simulink model "CryoDetMultiChan_CMB"  (R2016b)
settings: Solver=ode45  StartTime=0.0  StopTime=400e-6  MaxStep=Tclk/4  RelTol=1e-3
values from neighbouring files (symbols this model uses):
  ds_axi = 16    [setupCryoFPGA_CMB.m]
  Fclk = Fadc    (= 307200000)    [setupCryoFPGA_CMB.m]
  lpf = tf(num,den)    [setupCryoFPGA_CMB.m]
  Tclk = 1/Fclk    (= 3.25520833333e-09)    [setupCryoFPGA_CMB.m]
  Ts = 1/Fs    (= 3.25520833333e-09)    [setupADCtoDACloopback.m]    (also in setupCryoFPGA_CMB.m)
undefined symbols (not defined in the file or in its folder): AXI4, i, Lite, xlipgetpartsetting
libraries: xbsIndex_r4 x2215, hdlsllib x6, simulink x3, CryoDetLib x2
(part 4 of 16)

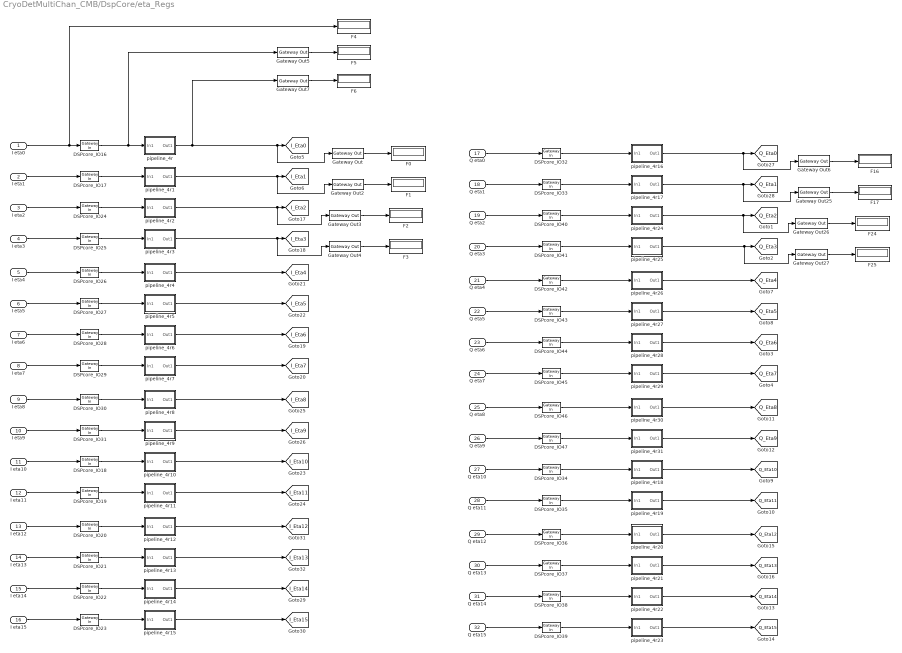
== system CryoDetMultiChan_CMB/DspCore/eta_Regs ==
  "I eta0 " : Inport
  I eta1 : Inport  Port=2
  I eta2 : Inport  Port=3
  I eta3 : Inport  Port=4
  I eta4 : Inport  Port=5
  I eta5 : Inport  Port=6
  I eta6 : Inport  Port=7
  I eta7 : Inport  Port=8
  I eta8 : Inport  Port=9
  I eta9 : Inport  Port=10
  I eta10 : Inport  Port=11
  I eta11 : Inport  Port=12
  I eta12 : Inport  Port=13
  I eta13 : Inport  Port=14
  I eta14 : Inport  Port=15
  I eta15 : Inport  Port=16
  Q eta0 : Inport  Port=17
  Q eta1 : Inport  Port=18
  Q eta2 : Inport  Port=19
  Q eta3 : Inport  Port=20
  Q eta4 : Inport  Port=21
  Q eta5 : Inport  Port=22
  Q eta6 : Inport  Port=23
  Q eta7 : Inport  Port=24
  Q eta8 : Inport  Port=25
  Q eta9 : Inport  Port=26
  Q eta10 : Inport  Port=27
  Q eta11 : Inport  Port=28
  Q eta12 : Inport  Port=29
  Q eta13 : Inport  Port=30
  Q eta14 : Inport  Port=31
  Q eta15 : Inport  Port=32
  DSPcore_IO16 : xbsIndex_r4/Gateway In  gui_display_data_type=Fixed-point  arith_type="Signed  (2's comp)"  n_bits=32  bin_pt=31  preci_type=Single  exp_width=8  frac_width=24  rows=1  columns=1  quantization=Truncate  overflow=Wrap  period=Tclk*ds_axi  UseAsADC=off  ADCChannel='1'  interface=AXI4-Lite  automatic_assignment=off  address_offset=hex2dec('A00')  intf_name=''  intf_description=''  default_value=0  timing_constraint=None  locs_specified=off  LOCs={}  io_standard={}  inherit_from_input=off  hdl_port=on  dbl_ovrd=off  block_type=gatewayin
  DSPcore_IO17 : xbsIndex_r4/Gateway In  gui_display_data_type=Fixed-point  arith_type="Signed  (2's comp)"  n_bits=32  bin_pt=31  preci_type=Single  exp_width=8  frac_width=24  rows=1  columns=1  quantization=Truncate  overflow=Wrap  period=Tclk*ds_axi  UseAsADC=off  ADCChannel='1'  interface=AXI4-Lite  automatic_assignment=off  address_offset=hex2dec('A08')  intf_name=''  intf_description=''  default_value=0  timing_constraint=None  locs_specified=off  LOCs={}  io_standard={}  inherit_from_input=off  hdl_port=on  dbl_ovrd=off  block_type=gatewayin
  DSPcore_IO18 : xbsIndex_r4/Gateway In  gui_display_data_type=Fixed-point  arith_type="Signed  (2's comp)"  n_bits=32  bin_pt=31  preci_type=Single  exp_width=8  frac_width=24  rows=1  columns=1  quantization=Truncate  overflow=Wrap  period=Tclk*ds_axi  UseAsADC=off  ADCChannel='1'  interface=AXI4-Lite  automatic_assignment=off  address_offset=hex2dec('A50')  intf_name=''  intf_description=''  default_value=0  timing_constraint=None  locs_specified=off  LOCs={}  io_standard={}  inherit_from_input=off  hdl_port=on  dbl_ovrd=off  block_type=gatewayin
  DSPcore_IO19 : xbsIndex_r4/Gateway In  gui_display_data_type=Fixed-point  arith_type="Signed  (2's comp)"  n_bits=32  bin_pt=31  preci_type=Single  exp_width=8  frac_width=24  rows=1  columns=1  quantization=Truncate  overflow=Wrap  period=Tclk*ds_axi  UseAsADC=off  ADCChannel='1'  interface=AXI4-Lite  automatic_assignment=off  address_offset=hex2dec('A58')  intf_name=''  intf_description=''  default_value=0  timing_constraint=None  locs_specified=off  LOCs={}  io_standard={}  inherit_from_input=off  hdl_port=on  dbl_ovrd=off  block_type=gatewayin
  DSPcore_IO20 : xbsIndex_r4/Gateway In  gui_display_data_type=Fixed-point  arith_type="Signed  (2's comp)"  n_bits=32  bin_pt=31  preci_type=Single  exp_width=8  frac_width=24  rows=1  columns=1  quantization=Truncate  overflow=Wrap  period=Tclk*ds_axi  UseAsADC=off  ADCChannel='1'  interface=AXI4-Lite  automatic_assignment=off  address_offset=hex2dec('A60')  intf_name=''  intf_description=''  default_value=0  timing_constraint=None  locs_specified=off  LOCs={}  io_standard={}  inherit_from_input=off  hdl_port=on  dbl_ovrd=off  block_type=gatewayin
  DSPcore_IO21 : xbsIndex_r4/Gateway In  gui_display_data_type=Fixed-point  arith_type="Signed  (2's comp)"  n_bits=32  bin_pt=31  preci_type=Single  exp_width=8  frac_width=24  rows=1  columns=1  quantization=Truncate  overflow=Wrap  period=Tclk*ds_axi  UseAsADC=off  ADCChannel='1'  interface=AXI4-Lite  automatic_assignment=off  address_offset=hex2dec('A68')  intf_name=''  intf_description=''  default_value=0  timing_constraint=None  locs_specified=off  LOCs={}  io_standard={}  inherit_from_input=off  hdl_port=on  dbl_ovrd=off  block_type=gatewayin
  DSPcore_IO22 : xbsIndex_r4/Gateway In  gui_display_data_type=Fixed-point  arith_type="Signed  (2's comp)"  n_bits=32  bin_pt=31  preci_type=Single  exp_width=8  frac_width=24  rows=1  columns=1  quantization=Truncate  overflow=Wrap  period=Tclk*ds_axi  UseAsADC=off  ADCChannel='1'  interface=AXI4-Lite  automatic_assignment=off  address_offset=hex2dec('A70')  intf_name=''  intf_description=''  default_value=0  timing_constraint=None  locs_specified=off  LOCs={}  io_standard={}  inherit_from_input=off  hdl_port=on  dbl_ovrd=off  block_type=gatewayin
  DSPcore_IO23 : xbsIndex_r4/Gateway In  gui_display_data_type=Fixed-point  arith_type="Signed  (2's comp)"  n_bits=32  bin_pt=31  preci_type=Single  exp_width=8  frac_width=24  rows=1  columns=1  quantization=Truncate  overflow=Wrap  period=Tclk*ds_axi  UseAsADC=off  ADCChannel='1'  interface=AXI4-Lite  automatic_assignment=off  address_offset=hex2dec('A78')  intf_name=''  intf_description=''  default_value=0  timing_constraint=None  locs_specified=off  LOCs={}  io_standard={}  inherit_from_input=off  hdl_port=on  dbl_ovrd=off  block_type=gatewayin
  DSPcore_IO24 : xbsIndex_r4/Gateway In  gui_display_data_type=Fixed-point  arith_type="Signed  (2's comp)"  n_bits=32  bin_pt=31  preci_type=Single  exp_width=8  frac_width=24  rows=1  columns=1  quantization=Truncate  overflow=Wrap  period=Tclk*ds_axi  UseAsADC=off  ADCChannel='1'  interface=AXI4-Lite  automatic_assignment=off  address_offset=hex2dec('A10')  intf_name=''  intf_description=''  default_value=0  timing_constraint=None  locs_specified=off  LOCs={}  io_standard={}  inherit_from_input=off  hdl_port=on  dbl_ovrd=off  block_type=gatewayin
  DSPcore_IO25 : xbsIndex_r4/Gateway In  gui_display_data_type=Fixed-point  arith_type="Signed  (2's comp)"  n_bits=32  bin_pt=31  preci_type=Single  exp_width=8  frac_width=24  rows=1  columns=1  quantization=Truncate  overflow=Wrap  period=Tclk*ds_axi  UseAsADC=off  ADCChannel='1'  interface=AXI4-Lite  automatic_assignment=off  address_offset=hex2dec('A18')  intf_name=''  intf_description=''  default_value=0  timing_constraint=None  locs_specified=off  LOCs={}  io_standard={}  inherit_from_input=off  hdl_port=on  dbl_ovrd=off  block_type=gatewayin
  DSPcore_IO26 : xbsIndex_r4/Gateway In  gui_display_data_type=Fixed-point  arith_type="Signed  (2's comp)"  n_bits=32  bin_pt=31  preci_type=Single  exp_width=8  frac_width=24  rows=1  columns=1  quantization=Truncate  overflow=Wrap  period=Tclk*ds_axi  UseAsADC=off  ADCChannel='1'  interface=AXI4-Lite  automatic_assignment=off  address_offset=hex2dec('A20')  intf_name=''  intf_description=''  default_value=0  timing_constraint=None  locs_specified=off  LOCs={}  io_standard={}  inherit_from_input=off  hdl_port=on  dbl_ovrd=off  block_type=gatewayin
  DSPcore_IO27 : xbsIndex_r4/Gateway In  gui_display_data_type=Fixed-point  arith_type="Signed  (2's comp)"  n_bits=32  bin_pt=31  preci_type=Single  exp_width=8  frac_width=24  rows=1  columns=1  quantization=Truncate  overflow=Wrap  period=Tclk*ds_axi  UseAsADC=off  ADCChannel='1'  interface=AXI4-Lite  automatic_assignment=off  address_offset=hex2dec('A28')  intf_name=''  intf_description=''  default_value=0  timing_constraint=None  locs_specified=off  LOCs={}  io_standard={}  inherit_from_input=off  hdl_port=on  dbl_ovrd=off  block_type=gatewayin
  DSPcore_IO28 : xbsIndex_r4/Gateway In  gui_display_data_type=Fixed-point  arith_type="Signed  (2's comp)"  n_bits=32  bin_pt=31  preci_type=Single  exp_width=8  frac_width=24  rows=1  columns=1  quantization=Truncate  overflow=Wrap  period=Tclk*ds_axi  UseAsADC=off  ADCChannel='1'  interface=AXI4-Lite  automatic_assignment=off  address_offset=hex2dec('A30')  intf_name=''  intf_description=''  default_value=0  timing_constraint=None  locs_specified=off  LOCs={}  io_standard={}  inherit_from_input=off  hdl_port=on  dbl_ovrd=off  block_type=gatewayin
  DSPcore_IO29 : xbsIndex_r4/Gateway In  gui_display_data_type=Fixed-point  arith_type="Signed  (2's comp)"  n_bits=32  bin_pt=31  preci_type=Single  exp_width=8  frac_width=24  rows=1  columns=1  quantization=Truncate  overflow=Wrap  period=Tclk*ds_axi  UseAsADC=off  ADCChannel='1'  interface=AXI4-Lite  automatic_assignment=off  address_offset=hex2dec('A38')  intf_name=''  intf_description=''  default_value=0  timing_constraint=None  locs_specified=off  LOCs={}  io_standard={}  inherit_from_input=off  hdl_port=on  dbl_ovrd=off  block_type=gatewayin
  DSPcore_IO30 : xbsIndex_r4/Gateway In  gui_display_data_type=Fixed-point  arith_type="Signed  (2's comp)"  n_bits=32  bin_pt=31  preci_type=Single  exp_width=8  frac_width=24  rows=1  columns=1  quantization=Truncate  overflow=Wrap  period=Tclk*ds_axi  UseAsADC=off  ADCChannel='1'  interface=AXI4-Lite  automatic_assignment=off  address_offset=hex2dec('A40')  intf_name=''  intf_description=''  default_value=0  timing_constraint=None  locs_specified=off  LOCs={}  io_standard={}  inherit_from_input=off  hdl_port=on  dbl_ovrd=off  block_type=gatewayin
  DSPcore_IO31 : xbsIndex_r4/Gateway In  gui_display_data_type=Fixed-point  arith_type="Signed  (2's comp)"  n_bits=32  bin_pt=31  preci_type=Single  exp_width=8  frac_width=24  rows=1  columns=1  quantization=Truncate  overflow=Wrap  period=Tclk*ds_axi  UseAsADC=off  ADCChannel='1'  interface=AXI4-Lite  automatic_assignment=off  address_offset=hex2dec('A48')  intf_name=''  intf_description=''  default_value=0  timing_constraint=None  locs_specified=off  LOCs={}  io_standard={}  inherit_from_input=off  hdl_port=on  dbl_ovrd=off  block_type=gatewayin
  DSPcore_IO32 : xbsIndex_r4/Gateway In  gui_display_data_type=Fixed-point  arith_type="Signed  (2's comp)"  n_bits=32  bin_pt=31  preci_type=Single  exp_width=8  frac_width=24  rows=1  columns=1  quantization=Truncate  overflow=Wrap  period=Tclk*ds_axi  UseAsADC=off  ADCChannel='1'  interface=AXI4-Lite  automatic_assignment=off  address_offset=hex2dec('A04')  intf_name=''  intf_description=''  default_value=0  timing_constraint=None  locs_specified=off  LOCs={}  io_standard={}  inherit_from_input=off  hdl_port=on  dbl_ovrd=off  block_type=gatewayin
  DSPcore_IO33 : xbsIndex_r4/Gateway In  gui_display_data_type=Fixed-point  arith_type="Signed  (2's comp)"  n_bits=32  bin_pt=31  preci_type=Single  exp_width=8  frac_width=24  rows=1  columns=1  quantization=Truncate  overflow=Wrap  period=Tclk*ds_axi  UseAsADC=off  ADCChannel='1'  interface=AXI4-Lite  automatic_assignment=off  address_offset=hex2dec('A0C')  intf_name=''  intf_description=''  default_value=0  timing_constraint=None  locs_specified=off  LOCs={}  io_standard={}  inherit_from_input=off  hdl_port=on  dbl_ovrd=off  block_type=gatewayin
  DSPcore_IO34 : xbsIndex_r4/Gateway In  gui_display_data_type=Fixed-point  arith_type="Signed  (2's comp)"  n_bits=32  bin_pt=31  preci_type=Single  exp_width=8  frac_width=24  rows=1  columns=1  quantization=Truncate  overflow=Wrap  period=Tclk*ds_axi  UseAsADC=off  ADCChannel='1'  interface=AXI4-Lite  automatic_assignment=off  address_offset=hex2dec('A54')  intf_name=''  intf_description=''  default_value=0  timing_constraint=None  locs_specified=off  LOCs={}  io_standard={}  inherit_from_input=off  hdl_port=on  dbl_ovrd=off  block_type=gatewayin
  DSPcore_IO35 : xbsIndex_r4/Gateway In  gui_display_data_type=Fixed-point  arith_type="Signed  (2's comp)"  n_bits=32  bin_pt=31  preci_type=Single  exp_width=8  frac_width=24  rows=1  columns=1  quantization=Truncate  overflow=Wrap  period=Tclk*ds_axi  UseAsADC=off  ADCChannel='1'  interface=AXI4-Lite  automatic_assignment=off  address_offset=hex2dec('A5C')  intf_name=''  intf_description=''  default_value=0  timing_constraint=None  locs_specified=off  LOCs={}  io_standard={}  inherit_from_input=off  hdl_port=on  dbl_ovrd=off  block_type=gatewayin
  DSPcore_IO36 : xbsIndex_r4/Gateway In  gui_display_data_type=Fixed-point  arith_type="Signed  (2's comp)"  n_bits=32  bin_pt=31  preci_type=Single  exp_width=8  frac_width=24  rows=1  columns=1  quantization=Truncate  overflow=Wrap  period=Tclk*ds_axi  UseAsADC=off  ADCChannel='1'  interface=AXI4-Lite  automatic_assignment=off  address_offset=hex2dec('A64')  intf_name=''  intf_description=''  default_value=0  timing_constraint=None  locs_specified=off  LOCs={}  io_standard={}  inherit_from_input=off  hdl_port=on  dbl_ovrd=off  block_type=gatewayin
  DSPcore_IO37 : xbsIndex_r4/Gateway In  gui_display_data_type=Fixed-point  arith_type="Signed  (2's comp)"  n_bits=32  bin_pt=31  preci_type=Single  exp_width=8  frac_width=24  rows=1  columns=1  quantization=Truncate  overflow=Wrap  period=Tclk*ds_axi  UseAsADC=off  ADCChannel='1'  interface=AXI4-Lite  automatic_assignment=off  address_offset=hex2dec('A6C')  intf_name=''  intf_description=''  default_value=0  timing_constraint=None  locs_specified=off  LOCs={}  io_standard={}  inherit_from_input=off  hdl_port=on  dbl_ovrd=off  block_type=gatewayin
  DSPcore_IO38 : xbsIndex_r4/Gateway In  gui_display_data_type=Fixed-point  arith_type="Signed  (2's comp)"  n_bits=32  bin_pt=31  preci_type=Single  exp_width=8  frac_width=24  rows=1  columns=1  quantization=Truncate  overflow=Wrap  period=Tclk*ds_axi  UseAsADC=off  ADCChannel='1'  interface=AXI4-Lite  automatic_assignment=off  address_offset=hex2dec('A74')  intf_name=''  intf_description=''  default_value=0  timing_constraint=None  locs_specified=off  LOCs={}  io_standard={}  inherit_from_input=off  hdl_port=on  dbl_ovrd=off  block_type=gatewayin
  DSPcore_IO39 : xbsIndex_r4/Gateway In  gui_display_data_type=Fixed-point  arith_type="Signed  (2's comp)"  n_bits=32  bin_pt=31  preci_type=Single  exp_width=8  frac_width=24  rows=1  columns=1  quantization=Truncate  overflow=Wrap  period=Tclk*ds_axi  UseAsADC=off  ADCChannel='1'  interface=AXI4-Lite  automatic_assignment=off  address_offset=hex2dec('A7C')  intf_name=''  intf_description=''  default_value=0  timing_constraint=None  locs_specified=off  LOCs={}  io_standard={}  inherit_from_input=off  hdl_port=on  dbl_ovrd=off  block_type=gatewayin
  DSPcore_IO40 : xbsIndex_r4/Gateway In  gui_display_data_type=Fixed-point  arith_type="Signed  (2's comp)"  n_bits=32  bin_pt=31  preci_type=Single  exp_width=8  frac_width=24  rows=1  columns=1  quantization=Truncate  overflow=Wrap  period=Tclk*ds_axi  UseAsADC=off  ADCChannel='1'  interface=AXI4-Lite  automatic_assignment=off  address_offset=hex2dec('A14')  intf_name=''  intf_description=''  default_value=0  timing_constraint=None  locs_specified=off  LOCs={}  io_standard={}  inherit_from_input=off  hdl_port=on  dbl_ovrd=off  block_type=gatewayin
  DSPcore_IO41 : xbsIndex_r4/Gateway In  gui_display_data_type=Fixed-point  arith_type="Signed  (2's comp)"  n_bits=32  bin_pt=31  preci_type=Single  exp_width=8  frac_width=24  rows=1  columns=1  quantization=Truncate  overflow=Wrap  period=Tclk*ds_axi  UseAsADC=off  ADCChannel='1'  interface=AXI4-Lite  automatic_assignment=off  address_offset=hex2dec('A1C')  intf_name=''  intf_description=''  default_value=0  timing_constraint=None  locs_specified=off  LOCs={}  io_standard={}  inherit_from_input=off  hdl_port=on  dbl_ovrd=off  block_type=gatewayin
  DSPcore_IO42 : xbsIndex_r4/Gateway In  gui_display_data_type=Fixed-point  arith_type="Signed  (2's comp)"  n_bits=32  bin_pt=31  preci_type=Single  exp_width=8  frac_width=24  rows=1  columns=1  quantization=Truncate  overflow=Wrap  period=Tclk*ds_axi  UseAsADC=off  ADCChannel='1'  interface=AXI4-Lite  automatic_assignment=off  address_offset=hex2dec('A24')  intf_name=''  intf_description=''  default_value=0  timing_constraint=None  locs_specified=off  LOCs={}  io_standard={}  inherit_from_input=off  hdl_port=on  dbl_ovrd=off  block_type=gatewayin
  DSPcore_IO43 : xbsIndex_r4/Gateway In  gui_display_data_type=Fixed-point  arith_type="Signed  (2's comp)"  n_bits=32  bin_pt=31  preci_type=Single  exp_width=8  frac_width=24  rows=1  columns=1  quantization=Truncate  overflow=Wrap  period=Tclk*ds_axi  UseAsADC=off  ADCChannel='1'  interface=AXI4-Lite  automatic_assignment=off  address_offset=hex2dec('A2C')  intf_name=''  intf_description=''  default_value=0  timing_constraint=None  locs_specified=off  LOCs={}  io_standard={}  inherit_from_input=off  hdl_port=on  dbl_ovrd=off  block_type=gatewayin
  DSPcore_IO44 : xbsIndex_r4/Gateway In  gui_display_data_type=Fixed-point  arith_type="Signed  (2's comp)"  n_bits=32  bin_pt=31  preci_type=Single  exp_width=8  frac_width=24  rows=1  columns=1  quantization=Truncate  overflow=Wrap  period=Tclk*ds_axi  UseAsADC=off  ADCChannel='1'  interface=AXI4-Lite  automatic_assignment=off  address_offset=hex2dec('A34')  intf_name=''  intf_description=''  default_value=0  timing_constraint=None  locs_specified=off  LOCs={}  io_standard={}  inherit_from_input=off  hdl_port=on  dbl_ovrd=off  block_type=gatewayin
  DSPcore_IO45 : xbsIndex_r4/Gateway In  gui_display_data_type=Fixed-point  arith_type="Signed  (2's comp)"  n_bits=32  bin_pt=31  preci_type=Single  exp_width=8  frac_width=24  rows=1  columns=1  quantization=Truncate  overflow=Wrap  period=Tclk*ds_axi  UseAsADC=off  ADCChannel='1'  interface=AXI4-Lite  automatic_assignment=off  address_offset=hex2dec('A3C')  intf_name=''  intf_description=''  default_value=0  timing_constraint=None  locs_specified=off  LOCs={}  io_standard={}  inherit_from_input=off  hdl_port=on  dbl_ovrd=off  block_type=gatewayin
  DSPcore_IO46 : xbsIndex_r4/Gateway In  gui_display_data_type=Fixed-point  arith_type="Signed  (2's comp)"  n_bits=32  bin_pt=31  preci_type=Single  exp_width=8  frac_width=24  rows=1  columns=1  quantization=Truncate  overflow=Wrap  period=Tclk*ds_axi  UseAsADC=off  ADCChannel='1'  interface=AXI4-Lite  automatic_assignment=off  address_offset=hex2dec('A44')  intf_name=''  intf_description=''  default_value=0  timing_constraint=None  locs_specified=off  LOCs={}  io_standard={}  inherit_from_input=off  hdl_port=on  dbl_ovrd=off  block_type=gatewayin
  DSPcore_IO47 : xbsIndex_r4/Gateway In  gui_display_data_type=Fixed-point  arith_type="Signed  (2's comp)"  n_bits=32  bin_pt=31  preci_type=Single  exp_width=8  frac_width=24  rows=1  columns=1  quantization=Truncate  overflow=Wrap  period=Tclk*ds_axi  UseAsADC=off  ADCChannel='1'  interface=AXI4-Lite  automatic_assignment=off  address_offset=hex2dec('A4C')  intf_name=''  intf_description=''  default_value=0  timing_constraint=None  locs_specified=off  LOCs={}  io_standard={}  inherit_from_input=off  hdl_port=on  dbl_ovrd=off  block_type=gatewayin
  F{0..6,16..17,24..25} (11 alike) : Display
  Gateway Out{,2..7,25..27} (10 alike) : xbsIndex_r4/Gateway Out  inherit_from_input=on  hdl_port=off  rows=1  columns=1  UseAsDAC=off  DACChannel='1'  interface=None  automatic_assignment=on  address_offset=hex2dec('00')  intf_name=''  intf_description=''  timing_constraint=None  locs_specified=off  LOCs={}  io_standard={}  block_type=gatewayout
  pipeline_4r : Subsystem
  pipeline_4r1 : Subsystem
  pipeline_4r10 : Subsystem
  pipeline_4r11 : Subsystem
  pipeline_4r12 : Subsystem
  pipeline_4r13 : Subsystem
  pipeline_4r14 : Subsystem
  pipeline_4r15 : Subsystem
  pipeline_4r16 : Subsystem
  pipeline_4r17 : Subsystem
  pipeline_4r18 : Subsystem
  pipeline_4r19 : Subsystem
  pipeline_4r2 : Subsystem
  pipeline_4r20 : Subsystem
  pipeline_4r21 : Subsystem
  pipeline_4r22 : Subsystem
  pipeline_4r23 : Subsystem
  pipeline_4r24 : Subsystem
  pipeline_4r25 : Subsystem
  pipeline_4r26 : Subsystem
  pipeline_4r27 : Subsystem
  pipeline_4r28 : Subsystem
  pipeline_4r29 : Subsystem
  pipeline_4r3 : Subsystem
  pipeline_4r30 : Subsystem
  pipeline_4r31 : Subsystem
  pipeline_4r4 : Subsystem
  pipeline_4r5 : Subsystem
  pipeline_4r6 : Subsystem
  pipeline_4r7 : Subsystem
  pipeline_4r8 : Subsystem
  pipeline_4r9 : Subsystem
  tag scope: I_Eta0=global, I_Eta10=global, I_Eta11=global, I_Eta12=global, I_Eta13=global, I_Eta14=global, I_Eta15=global, I_Eta1=global, I_Eta2=global, I_Eta3=global, I_Eta4=global, I_Eta5=global, I_Eta6=global, I_Eta7=global, I_Eta8=global, I_Eta9=global, Q_Eta0=global, Q_Eta10=global, Q_Eta11=global, Q_Eta12=global, Q_Eta13=global, Q_Eta14=global, Q_Eta15=global, Q_Eta1=global, Q_Eta2=global, Q_Eta3=global, Q_Eta4=global, Q_Eta5=global, Q_Eta6=global, Q_Eta7=global, Q_Eta8=global, Q_Eta9=global
  wires:
  I eta14/1 -> DSPcore_IO22/1
  pipeline_4r4/1(Out1) -> [I_Eta4]
  DSPcore_IO26/1 -> pipeline_4r4/1(In1)
  DSPcore_IO21/1 -> pipeline_4r13/1(In1)
  I eta13/1 -> DSPcore_IO21/1
  DSPcore_IO27/1 -> pipeline_4r5/1(In1)
  I eta15/1 -> DSPcore_IO23/1
  DSPcore_IO18/1 -> pipeline_4r10/1(In1)
  I eta7/1 -> DSPcore_IO29/1
  I eta11/1 -> DSPcore_IO19/1
  I eta9/1 -> DSPcore_IO31/1
  Gateway Out4/1 -> F3/1
  DSPcore_IO25/1 -> pipeline_4r3/1(In1)
  I eta5/1 -> DSPcore_IO27/1
  pipeline_4r5/1(Out1) -> [I_Eta5]
  I eta8/1 -> DSPcore_IO30/1
  DSPcore_IO20/1 -> pipeline_4r12/1(In1)
  I eta4/1 -> DSPcore_IO26/1
  Gateway Out2/1 -> F1/1
  pipeline_4r1/1(Out1) -> [I_Eta1], Gateway Out2/1
  DSPcore_IO19/1 -> pipeline_4r11/1(In1)
  DSPcore_IO23/1 -> pipeline_4r15/1(In1)
  I eta10/1 -> DSPcore_IO18/1
  I eta2/1 -> DSPcore_IO24/1
  Gateway Out3/1 -> F2/1
  DSPcore_IO24/1 -> pipeline_4r2/1(In1)
  DSPcore_IO17/1 -> pipeline_4r1/1(In1)
  I eta1/1 -> DSPcore_IO17/1
  DSPcore_IO30/1 -> pipeline_4r8/1(In1)
  DSPcore_IO22/1 -> pipeline_4r14/1(In1)
  I eta6/1 -> DSPcore_IO28/1
  I eta3/1 -> DSPcore_IO25/1
  Gateway Out/1 -> F0/1
  pipeline_4r/1(Out1) -> [I_Eta0], Gateway Out/1, Gateway Out7/1
  DSPcore_IO16/1 -> Gateway Out5/1, pipeline_4r/1(In1)
  pipeline_4r6/1(Out1) -> [I_Eta6]
  DSPcore_IO29/1 -> pipeline_4r7/1(In1)
  I eta12/1 -> DSPcore_IO20/1
  DSPcore_IO28/1 -> pipeline_4r6/1(In1)
  Q eta14/1 -> DSPcore_IO38/1
  DSPcore_IO42/1 -> pipeline_4r26/1(In1)
  DSPcore_IO37/1 -> pipeline_4r21/1(In1)
  Q eta13/1 -> DSPcore_IO37/1
  Q eta15/1 -> DSPcore_IO39/1
  DSPcore_IO34/1 -> pipeline_4r18/1(In1)
  Q eta7/1 -> DSPcore_IO45/1
  Q eta11/1 -> DSPcore_IO35/1
  Q eta9/1 -> DSPcore_IO47/1
  Gateway Out27/1 -> F25/1
  DSPcore_IO41/1 -> pipeline_4r25/1(In1)
  Q eta5/1 -> DSPcore_IO43/1
  DSPcore_IO43/1 -> pipeline_4r27/1(In1)
  Q eta8/1 -> DSPcore_IO46/1
  DSPcore_IO36/1 -> pipeline_4r20/1(In1)
  Q eta4/1 -> DSPcore_IO42/1
  Gateway Out25/1 -> F17/1
  DSPcore_IO33/1 -> pipeline_4r17/1(In1)
  DSPcore_IO35/1 -> pipeline_4r19/1(In1)
  DSPcore_IO39/1 -> pipeline_4r23/1(In1)
  Q eta10/1 -> DSPcore_IO34/1
  DSPcore_IO47/1 -> pipeline_4r31/1(In1)
  Q eta2/1 -> DSPcore_IO40/1
  Gateway Out26/1 -> F24/1
  DSPcore_IO40/1 -> pipeline_4r24/1(In1)
  Q eta1/1 -> DSPcore_IO33/1
  DSPcore_IO46/1 -> pipeline_4r30/1(In1)
  DSPcore_IO38/1 -> pipeline_4r22/1(In1)
  Q eta6/1 -> DSPcore_IO44/1
  Q eta3/1 -> DSPcore_IO41/1
  Q eta0/1 -> DSPcore_IO32/1
  Gateway Out6/1 -> F16/1
  DSPcore_IO32/1 -> pipeline_4r16/1(In1)
  DSPcore_IO45/1 -> pipeline_4r29/1(In1)
  Q eta12/1 -> DSPcore_IO36/1
  DSPcore_IO44/1 -> pipeline_4r28/1(In1)
  Gateway Out5/1 -> F5/1
  Gateway Out7/1 -> F6/1
  "I eta0 "/1 -> F4/1, DSPcore_IO16/1
  DSPcore_IO31/1 -> pipeline_4r9/1(In1)
  pipeline_4r2/1(Out1) -> [I_Eta2], Gateway Out3/1
  pipeline_4r3/1(Out1) -> [I_Eta3], Gateway Out4/1
  pipeline_4r7/1(Out1) -> [I_Eta7]
  pipeline_4r12/1(Out1) -> [I_Eta12]
  pipeline_4r14/1(Out1) -> [I_Eta14]
  pipeline_4r13/1(Out1) -> [I_Eta13]
  pipeline_4r10/1(Out1) -> [I_Eta10]
  pipeline_4r11/1(Out1) -> [I_Eta11]
  pipeline_4r9/1(Out1) -> [I_Eta9]
  pipeline_4r15/1(Out1) -> [I_Eta15]
  pipeline_4r8/1(Out1) -> [I_Eta8]
  pipeline_4r21/1(Out1) -> [Q_Eta13]
  pipeline_4r22/1(Out1) -> [Q_Eta14]
  pipeline_4r23/1(Out1) -> [Q_Eta15]
  pipeline_4r24/1(Out1) -> [Q_Eta2], Gateway Out26/1
  pipeline_4r25/1(Out1) -> [Q_Eta3], Gateway Out27/1
  pipeline_4r26/1(Out1) -> [Q_Eta4]
  pipeline_4r17/1(Out1) -> [Q_Eta1], Gateway Out25/1
  pipeline_4r18/1(Out1) -> [Q_Eta10]
  pipeline_4r16/1(Out1) -> [Q_Eta0], Gateway Out6/1
  pipeline_4r29/1(Out1) -> [Q_Eta7]
  pipeline_4r27/1(Out1) -> [Q_Eta5]
  pipeline_4r28/1(Out1) -> [Q_Eta6]
  pipeline_4r30/1(Out1) -> [Q_Eta8]
  pipeline_4r31/1(Out1) -> [Q_Eta9]
  pipeline_4r19/1(Out1) -> [Q_Eta11]
  pipeline_4r20/1(Out1) -> [Q_Eta12]

== system CryoDetMultiChan_CMB/complex Notch0/imNotch ==
  note: Notch Filter with center angular frequency w, finite Q, and depth -26 dB
  In : Inport
  w0 : Inport  Port=2
  1/Q : Inport  Port=3
  Gain : Gain  Gain=.90
  Integrator1 : Integrator
  Integrator4 : Integrator
  Mult : Product
  Product : Product
  Product1 : Product
  Sum1 : Sum  Inputs=++|
  Sum2 : Sum  Inputs=|+-
  Sum3 : Sum  Inputs=-+|
  outt : Outport
  wires:
  w0/1 -> Product1/1, Product/1
  Integrator1/1 -> Product/2
  Product/1 -> Mult/1, Integrator4/1
  Integrator4/1 -> Product1/2
  1/Q/1 -> Mult/2
  Sum2/1 -> Integrator1/1
  In/1 -> Sum3/2, Sum2/1
  Sum1/1 -> Sum2/2
  Product1/1 -> Sum1/2
  Mult/1 -> Gain/1, Sum1/1
  Sum3/1 -> outt/1
  Gain/1 -> Sum3/1

== system CryoDetMultiChan_CMB/complex Notch0/reNotch ==
  note: Notch Filter with center angular frequency w, finite Q, and depth -26 dB
  In : Inport
  w0 : Inport  Port=2
  1/Q : Inport  Port=3
  Gain : Gain  Gain=.90
  Integrator1 : Integrator
  Integrator4 : Integrator
  Mult : Product
  Product : Product
  Product1 : Product
  Sum1 : Sum  Inputs=++|
  Sum2 : Sum  Inputs=|+-
  Sum3 : Sum  Inputs=-+|
  outt : Outport
  wires:
  w0/1 -> Product1/1, Product/1
  Integrator1/1 -> Product/2
  Product/1 -> Mult/1, Integrator4/1
  Integrator4/1 -> Product1/2
  1/Q/1 -> Mult/2
  Sum2/1 -> Integrator1/1
  In/1 -> Sum3/2, Sum2/1
  Sum1/1 -> Sum2/2
  Product1/1 -> Sum1/2
  Mult/1 -> Gain/1, Sum1/1
  Sum3/1 -> outt/1
  Gain/1 -> Sum3/1

== system CryoDetMultiChan_CMB/complex Notch1/imNotch ==
  note: Notch Filter with center angular frequency w, finite Q, and depth -26 dB
  In : Inport
  w0 : Inport  Port=2
  1/Q : Inport  Port=3
  Gain : Gain  Gain=.90
  Integrator1 : Integrator
  Integrator4 : Integrator
  Mult : Product
  Product : Product
  Product1 : Product
  Sum1 : Sum  Inputs=++|
  Sum2 : Sum  Inputs=|+-
  Sum3 : Sum  Inputs=-+|
  outt : Outport
  wires:
  w0/1 -> Product1/1, Product/1
  Integrator1/1 -> Product/2
  Product/1 -> Mult/1, Integrator4/1
  Integrator4/1 -> Product1/2
  1/Q/1 -> Mult/2
  Sum2/1 -> Integrator1/1
  In/1 -> Sum3/2, Sum2/1
  Sum1/1 -> Sum2/2
  Product1/1 -> Sum1/2
  Mult/1 -> Gain/1, Sum1/1
  Sum3/1 -> outt/1
  Gain/1 -> Sum3/1

== system CryoDetMultiChan_CMB/complex Notch1/reNotch ==
  note: Notch Filter with center angular frequency w, finite Q, and depth -26 dB
  In : Inport
  w0 : Inport  Port=2
  1/Q : Inport  Port=3
  Gain : Gain  Gain=.90
  Integrator1 : Integrator
  Integrator4 : Integrator
  Mult : Product
  Product : Product
  Product1 : Product
  Sum1 : Sum  Inputs=++|
  Sum2 : Sum  Inputs=|+-
  Sum3 : Sum  Inputs=-+|
  outt : Outport
  wires:
  w0/1 -> Product1/1, Product/1
  Integrator1/1 -> Product/2
  Product/1 -> Mult/1, Integrator4/1
  Integrator4/1 -> Product1/2
  1/Q/1 -> Mult/2
  Sum2/1 -> Integrator1/1
  In/1 -> Sum3/2, Sum2/1
  Sum1/1 -> Sum2/2
  Product1/1 -> Sum1/2
  Mult/1 -> Gain/1, Sum1/1
  Sum3/1 -> outt/1
  Gain/1 -> Sum3/1

== system CryoDetMultiChan_CMB/DspCore/DAC_fs_LO_Regs/pipeline_2r ==
  In1 : Inport
  Register2 : xbsIndex_r4/Register  init=0  rst=off  en=off  dbl_ovrd=off  block_type=register
  Register3 : xbsIndex_r4/Register  init=0  rst=off  en=off  dbl_ovrd=off  block_type=register
  Out1 : Outport
  wires:
  In1/1 -> Register2/1
  Register2/1 -> Register3/1
  Register3/1 -> Out1/1

== system CryoDetMultiChan_CMB/DspCore/DAC_fs_LO_Regs/pipeline_2r1 ==
  In1 : Inport
  Register2 : xbsIndex_r4/Register  init=0  rst=off  en=off  dbl_ovrd=off  block_type=register
  Register3 : xbsIndex_r4/Register  init=0  rst=off  en=off  dbl_ovrd=off  block_type=register
  Out1 : Outport
  wires:
  In1/1 -> Register2/1
  Register2/1 -> Register3/1
  Register3/1 -> Out1/1

== system CryoDetMultiChan_CMB/DspCore/DAC_fs_LO_Regs/pipeline_2r10 ==
  In1 : Inport
  Register2 : xbsIndex_r4/Register  init=0  rst=off  en=off  dbl_ovrd=off  block_type=register
  Register3 : xbsIndex_r4/Register  init=0  rst=off  en=off  dbl_ovrd=off  block_type=register
  Out1 : Outport
  wires:
  In1/1 -> Register2/1
  Register2/1 -> Register3/1
  Register3/1 -> Out1/1

== system CryoDetMultiChan_CMB/DspCore/DAC_fs_LO_Regs/pipeline_2r11 ==
  In1 : Inport
  Register2 : xbsIndex_r4/Register  init=0  rst=off  en=off  dbl_ovrd=off  block_type=register
  Register3 : xbsIndex_r4/Register  init=0  rst=off  en=off  dbl_ovrd=off  block_type=register
  Out1 : Outport
  wires:
  In1/1 -> Register2/1
  Register2/1 -> Register3/1
  Register3/1 -> Out1/1

== system CryoDetMultiChan_CMB/DspCore/DAC_fs_LO_Regs/pipeline_2r12 ==
  In1 : Inport
  Register2 : xbsIndex_r4/Register  init=0  rst=off  en=off  dbl_ovrd=off  block_type=register
  Register3 : xbsIndex_r4/Register  init=0  rst=off  en=off  dbl_ovrd=off  block_type=register
  Out1 : Outport
  wires:
  In1/1 -> Register2/1
  Register2/1 -> Register3/1
  Register3/1 -> Out1/1

== system CryoDetMultiChan_CMB/DspCore/DAC_fs_LO_Regs/pipeline_2r13 ==
  In1 : Inport
  Register2 : xbsIndex_r4/Register  init=0  rst=off  en=off  dbl_ovrd=off  block_type=register
  Register3 : xbsIndex_r4/Register  init=0  rst=off  en=off  dbl_ovrd=off  block_type=register
  Out1 : Outport
  wires:
  In1/1 -> Register2/1
  Register2/1 -> Register3/1
  Register3/1 -> Out1/1

== system CryoDetMultiChan_CMB/DspCore/DAC_fs_LO_Regs/pipeline_2r14 ==
  In1 : Inport
  Register2 : xbsIndex_r4/Register  init=0  rst=off  en=off  dbl_ovrd=off  block_type=register
  Register3 : xbsIndex_r4/Register  init=0  rst=off  en=off  dbl_ovrd=off  block_type=register
  Out1 : Outport
  wires:
  In1/1 -> Register2/1
  Register2/1 -> Register3/1
  Register3/1 -> Out1/1

== system CryoDetMultiChan_CMB/DspCore/DAC_fs_LO_Regs/pipeline_2r15 ==
  In1 : Inport
  Register2 : xbsIndex_r4/Register  init=0  rst=off  en=off  dbl_ovrd=off  block_type=register
  Register3 : xbsIndex_r4/Register  init=0  rst=off  en=off  dbl_ovrd=off  block_type=register
  Out1 : Outport
  wires:
  In1/1 -> Register2/1
  Register2/1 -> Register3/1
  Register3/1 -> Out1/1

== system CryoDetMultiChan_CMB/DspCore/DAC_fs_LO_Regs/pipeline_2r2 ==
  In1 : Inport
  Register2 : xbsIndex_r4/Register  init=0  rst=off  en=off  dbl_ovrd=off  block_type=register
  Register3 : xbsIndex_r4/Register  init=0  rst=off  en=off  dbl_ovrd=off  block_type=register
  Out1 : Outport
  wires:
  In1/1 -> Register2/1
  Register2/1 -> Register3/1
  Register3/1 -> Out1/1

== system CryoDetMultiChan_CMB/DspCore/DAC_fs_LO_Regs/pipeline_2r3 ==
  In1 : Inport
  Register2 : xbsIndex_r4/Register  init=0  rst=off  en=off  dbl_ovrd=off  block_type=register
  Register3 : xbsIndex_r4/Register  init=0  rst=off  en=off  dbl_ovrd=off  block_type=register
  Out1 : Outport
  wires:
  In1/1 -> Register2/1
  Register2/1 -> Register3/1
  Register3/1 -> Out1/1

== system CryoDetMultiChan_CMB/DspCore/DAC_fs_LO_Regs/pipeline_2r4 ==
  In1 : Inport
  Register2 : xbsIndex_r4/Register  init=0  rst=off  en=off  dbl_ovrd=off  block_type=register
  Register3 : xbsIndex_r4/Register  init=0  rst=off  en=off  dbl_ovrd=off  block_type=register
  Out1 : Outport
  wires:
  In1/1 -> Register2/1
  Register2/1 -> Register3/1
  Register3/1 -> Out1/1

== system CryoDetMultiChan_CMB/DspCore/DAC_fs_LO_Regs/pipeline_2r5 ==
  In1 : Inport
  Register2 : xbsIndex_r4/Register  init=0  rst=off  en=off  dbl_ovrd=off  block_type=register
  Register3 : xbsIndex_r4/Register  init=0  rst=off  en=off  dbl_ovrd=off  block_type=register
  Out1 : Outport
  wires:
  In1/1 -> Register2/1
  Register2/1 -> Register3/1
  Register3/1 -> Out1/1

== system CryoDetMultiChan_CMB/DspCore/DAC_fs_LO_Regs/pipeline_2r6 ==
  In1 : Inport
  Register2 : xbsIndex_r4/Register  init=0  rst=off  en=off  dbl_ovrd=off  block_type=register
  Register3 : xbsIndex_r4/Register  init=0  rst=off  en=off  dbl_ovrd=off  block_type=register
  Out1 : Outport
  wires:
  In1/1 -> Register2/1
  Register2/1 -> Register3/1
  Register3/1 -> Out1/1

== system CryoDetMultiChan_CMB/DspCore/DAC_fs_LO_Regs/pipeline_2r7 ==
  In1 : Inport
  Register2 : xbsIndex_r4/Register  init=0  rst=off  en=off  dbl_ovrd=off  block_type=register
  Register3 : xbsIndex_r4/Register  init=0  rst=off  en=off  dbl_ovrd=off  block_type=register
  Out1 : Outport
  wires:
  In1/1 -> Register2/1
  Register2/1 -> Register3/1
  Register3/1 -> Out1/1

== system CryoDetMultiChan_CMB/DspCore/DAC_fs_LO_Regs/pipeline_2r8 ==
  In1 : Inport
  Register2 : xbsIndex_r4/Register  init=0  rst=off  en=off  dbl_ovrd=off  block_type=register
  Register3 : xbsIndex_r4/Register  init=0  rst=off  en=off  dbl_ovrd=off  block_type=register
  Out1 : Outport
  wires:
  In1/1 -> Register2/1
  Register2/1 -> Register3/1
  Register3/1 -> Out1/1

== system CryoDetMultiChan_CMB/DspCore/DAC_fs_LO_Regs/pipeline_2r9 ==
  In1 : Inport
  Register2 : xbsIndex_r4/Register  init=0  rst=off  en=off  dbl_ovrd=off  block_type=register
  Register3 : xbsIndex_r4/Register  init=0  rst=off  en=off  dbl_ovrd=off  block_type=register
  Out1 : Outport
  wires:
  In1/1 -> Register2/1
  Register2/1 -> Register3/1
  Register3/1 -> Out1/1

== system CryoDetMultiChan_CMB/DspCore/FTA_Ch0/ADC_IQ_Swap ==
  note: BAND 1 Input
  note: I & Q Swap Logic
      |
      | Added b/c I'm not sure how the ADC
      | actually maps the I & Q data onto the 32-b word
      | Once we work this out, it can be hard-wired
  Swap_en : Inport
  ADC_in : Inport  Port=2
  BitBasher : xbsIndex_r4/BitBasher  bitexpr=|  display_expr=on  sr_1=I  arith_type1="Signed  (2's comp)"  bin_pt1=15  sr_2=Q  arith_type2="Signed  (2's comp)"  bin_pt2=15  sr_3=3  arith_type3=Unsigned  bin_pt3=0  sr_4=4  arith_type4=Unsigned  bin_pt4=0  dbl_ovrd=off  block_type=bitbasher
      | I = {a[15:0]}
      | Q = {a[31:16]}
  Mux8 : xbsIndex_r4/Mux  inputs=2  en=off  latency=1  precision=Full  arith_type=Unsigned  n_bits=16  bin_pt=14  quantization=Truncate  overflow=Wrap  dbl_ovrd=off  block_type=mux
  Mux9 : xbsIndex_r4/Mux  inputs=2  en=off  latency=1  precision=Full  arith_type=Unsigned  n_bits=16  bin_pt=14  quantization=Truncate  overflow=Wrap  dbl_ovrd=off  block_type=mux
  ADC_I_out : Outport
  ADC_Q_out : Outport  Port=2
  wires:
  Mux8/1 -> ADC_I_out/1
  ADC_in/1 -> BitBasher/1
  Swap_en/1 -> Mux8/1, Mux9/1
  BitBasher/1 -> Mux9/3, Mux8/2
  BitBasher/2 -> Mux9/2, Mux8/3
  Mux9/1 -> ADC_Q_out/1

== system CryoDetMultiChan_CMB/DspCore/FTA_Ch0/DAC_Output_Fmt ==
  In1 : Inport
  BitBasher : xbsIndex_r4/BitBasher  bitexpr=|  display_expr=off  sr_1=DAC_Q  arith_type1=Unsigned  bin_pt1=0  sr_2=DAC_I  arith_type2=Unsigned  bin_pt2=0  sr_3=3  arith_type3=Unsigned  bin_pt3=0  sr_4=4  arith_type4=Unsigned  bin_pt4=0  dbl_ovrd=off  block_type=bitbasher
      | DAC_Q={Q[15:0],Qp[15:0]}
      | DAC_I={I[15:0],Ip[15:0]}
  Bus Selector : BusSelector  OutputSignals=DAC_out_Q,DAC_out_I,DAC_out_Qp,DAC_out_Ip
  Out_Q : Outport
  Out_I : Outport  Port=2
  wires:
  BitBasher/2 -> Out_I/1
  Bus Selector/2 -> BitBasher/2  "<DAC_out_I>"
  In1/1 -> Bus Selector/1
  Bus Selector/1 -> BitBasher/1  "<DAC_out_Q>"
  BitBasher/1 -> Out_Q/1
  Bus Selector/4 -> BitBasher/4  "<DAC_out_Ip>"
  Bus Selector/3 -> BitBasher/3  "<DAC_out_Qp>"

== system CryoDetMultiChan_CMB/DspCore/FTA_Ch0/RF switch ==
  note: Enable/disable RF
  note: To DAC
  note: From tone generators
  note: To Ref
  In1 : Inport
  Bus Creator : BusCreator  Inputs=4
  Bus Creator1 : BusCreator  Inputs=2
  Bus Selector : BusSelector  OutputSignals=Q sum,I sum,Qp sum,Ip sum
  Constant2 : xbsIndex_r4/Constant  const=0  gui_display_data_type=Fixed-point  arith_type=Signed (2's comp)  n_bits=16  bin_pt=15  preci_type=Single  exp_width=8  frac_width=24  explicit_period=off  period=1  equ=P=C  opselect=C  inp2=PCIN>>17  opr=+  inp1=P  carry=CIN  dbl_ovrd=off  block_type=constant
  Mux{1..4} (4 alike) : xbsIndex_r4/Mux  inputs=2  en=off  latency=1  precision=User Defined  arith_type="Signed  (2's comp)"  n_bits=16  bin_pt=15  quantization=Truncate  overflow=Flag as error  dbl_ovrd=off  block_type=mux
  RF switch scope : Scope  NumInputPorts=5
  to_DAC : Outport
  to_REF : Outport  Port=2
  wires:
  [RFen] -> RF switch scope/1, Mux3/1, Mux4/1, Mux1/1, Mux2/1
  Constant2/1 -> Mux4/2, Mux3/2, Mux1/2, Mux2/2
  Bus Creator/1 -> to_DAC/1
  In1/1 -> Bus Selector/1
  Mux2/1 -> Bus Creator1/1, Bus Creator/1  "DAC_Q"
  Mux1/1 -> Bus Creator1/2, Bus Creator/2, RF switch scope/4  "DAC_I"
  Mux4/1 -> Bus Creator/3  "DAC_Qp"
  Mux3/1 -> RF switch scope/5, Bus Creator/4  "DAC_Ip"
  Bus Selector/1 -> Mux2/3  "<Q sum>"
  Bus Selector/2 -> RF switch scope/2, Mux1/3  "<I sum>"
  Bus Selector/3 -> Mux4/3  "<Qp sum>"
  Bus Selector/4 -> RF switch scope/3, Mux3/3  "<Ip sum>"
  Bus Creator1/1 -> to_REF/1

== system CryoDetMultiChan_CMB/DspCore/FTA_Ch0/Ref Delay ==
  note: Delays DAC output data used as Reference for input signal
      | Delay is to compensate for delay of DAC (big), up/downconverter, cable plant, cryostat etc.
      | This is to prevent too much delay mismatch from winding up phase vs. frequency of S21's of sidebands wrt to central line
  In1 : Inport
  Addressable Shift Register : xbsIndex_r4/Addressable Shift Register  infer_latency=on  depth=2  initVector=[0]  en=off  use_behavioral_HDL=on  Optimization=Resource  dbl_ovrd=off  block_type=addrsr
      settings: infoedit="Delay of configurable length.  Any element in the delay line can be addressed and driven onto the output port.<br><br>Hardware notes: Generates fast, compact FIFO-style shift registers or delay lines using SRL16/SRL32 mode of the slice LUTs"
  Addressable Shift Register1 : xbsIndex_r4/Addressable Shift Register  infer_latency=on  depth=2  initVector=[0]  en=off  use_behavioral_HDL=on  Optimization=Resource  dbl_ovrd=off  block_type=addrsr
      settings: infoedit="Delay of configurable length.  Any element in the delay line can be addressed and driven onto the output port.<br><br>Hardware notes: Generates fast, compact FIFO-style shift registers or delay lines using SRL16/SRL32 mode of the slice LUTs"
  Bus Selector : BusSelector  OutputSignals=DAC_Q,DAC_I
  Display : Display
      settings: Decimation=128
  Gateway Out : xbsIndex_r4/Gateway Out  inherit_from_input=off  hdl_port=off  rows=1  columns=1  UseAsDAC=off  DACChannel='1'  interface=None  automatic_assignment=on  address_offset=hex2dec('00')  intf_name=''  intf_description=''  timing_constraint=None  locs_specified=off  LOCs={}  io_standard={}  block_type=gatewayout
  Out_Q : Outport
  Out_I : Outport  Port=2
  wires:
  In1/1 -> Bus Selector/1
  Bus Selector/2 -> Addressable Shift Register1/1  "<DAC_I>"
  Bus Selector/1 -> Addressable Shift Register/1  "<DAC_Q>"
  Gateway Out/1 -> Display/1
  Addressable Shift Register/1 -> Out_Q/1
  Addressable Shift Register1/1 -> Out_I/1
  [refDel] -> Addressable Shift Register1/2, Addressable Shift Register/2, Gateway Out/1
